simulink model "olapfilt"  (Simulink 8.3)
settings: Solver=FixedStepDiscrete  SolverMode=SingleTasking  StartTime=0.0  StopTime=0.05  RelTol=1e-3  AbsTol=1e-6
libraries: dsparch4 x3, dspmisc x1, dspsrcs4 x1
settings Model: FPTRunName=Active  Creator=The MathWorks Inc.  CovMetricSettings=d  ExtModeTrigMode=oneshot  ExtModeArmWhenConnect=off
settings DataIOCC: LimitDataPoints=off  SaveOutput=off  SaveTime=off
settings OptimizationCC: BlockReduction=off  BooleanDataType=off  ExpressionDepthLimit=2147483647  RollThreshold=2  InitFltsAndDblsToZero=on
settings DebuggingCC: SaveWithParameterizedLinksMsg=none  SignalResolutionControl=TryResolveAllWithWarning  SolverPrmCheckMsg=none  MultiTaskDSMMsg=warning  MultiTaskCondExecSysMsg=none  IntegerOverflowMsg=none  FcnCallInpInsideContextMsg=UseLocalSettings  StrictBusMsg=None
settings RTWCC: IncludeERTFirstTime=on
settings GRTTargetCC: TargetFcnLib=ansi_tfl_tmw.mat

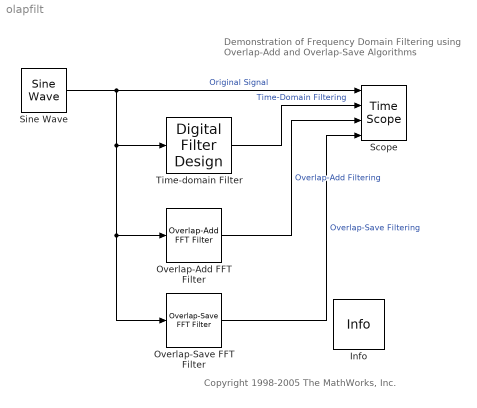
== system olapfilt ==
  note: Demonstration of Frequency Domain Filtering
      | using Overlap-Add and Overlap-Save Algorithms
  note: Copyright 1998-2005 The MathWorks, Inc.
  Info : dspmisc/Info  SystemSampleTime=-1
  Overlap-Add FFT Filter : dsparch4/Overlap-Add FFT Filter  Nfft=64  h=fir1(20,0.2)  output_complexity=Real  TreatMby1Signals=One channel
  Overlap-Save FFT Filter : dsparch4/Overlap-Save FFT Filter  nfft_in=64  h=fir1(20,0.2)  output_complexity=Real  TreatMby1Signals=One channel
  Scope : TimeScope  NumInputPorts=4  DefaultConfigurationName=spbscopes.TimeScopeBlockCfg  ScopeSpecification=DataTag2
  Sine Wave : dspsrcs4/Sine Wave  Amplitude=1  Frequency=500  Phase=0  SampleMode=Discrete  OutComplex=Real  CompMethod=Trigonometric fcn  TableSize=Speed  SampleTime=1/5000  SamplesPerFrame=1  ResetState=Restart at time zero  dataType=double  wordLen=16  udDataType=sfix(16)  fracBitsMode=Best precision  numFracBits=15  OutDataTypeStr=double  LastOutDataTypeStr=double
  Time-domain Filter : dsparch4/Digital Filter Design  mwdsp_browser_bugfix_var=off
  wires:
  Sine Wave/1 -> Time-domain Filter/1, Overlap-Add FFT Filter/1, Overlap-Save FFT Filter/1, Scope/1  "Original Signal"
  Time-domain Filter/1 -> Scope/2  "Time-Domain Filtering"
  Overlap-Add FFT Filter/1 -> Scope/3  "Overlap-Add Filtering"
  Overlap-Save FFT Filter/1 -> Scope/4  "Overlap-Save Filtering"
